simulink model "outdoor_weather_station"  (R2021b)
settings: Solver=VariableStepAuto  StartTime=0.0  StopTime=10.0  RelTol=1e-3
settings Model: Creator=solar  LastModifiedBy=solar

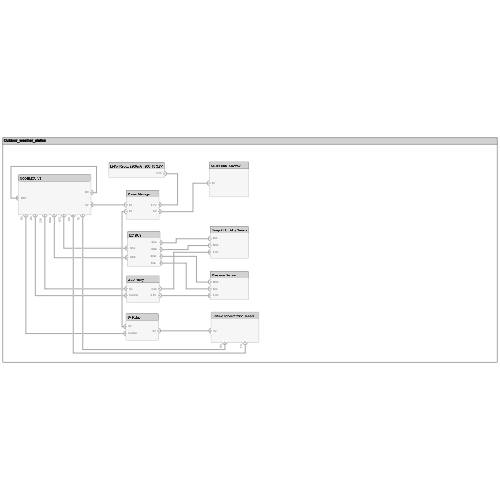
[thumbnail: Simulink's stored preview of the top-level diagram]
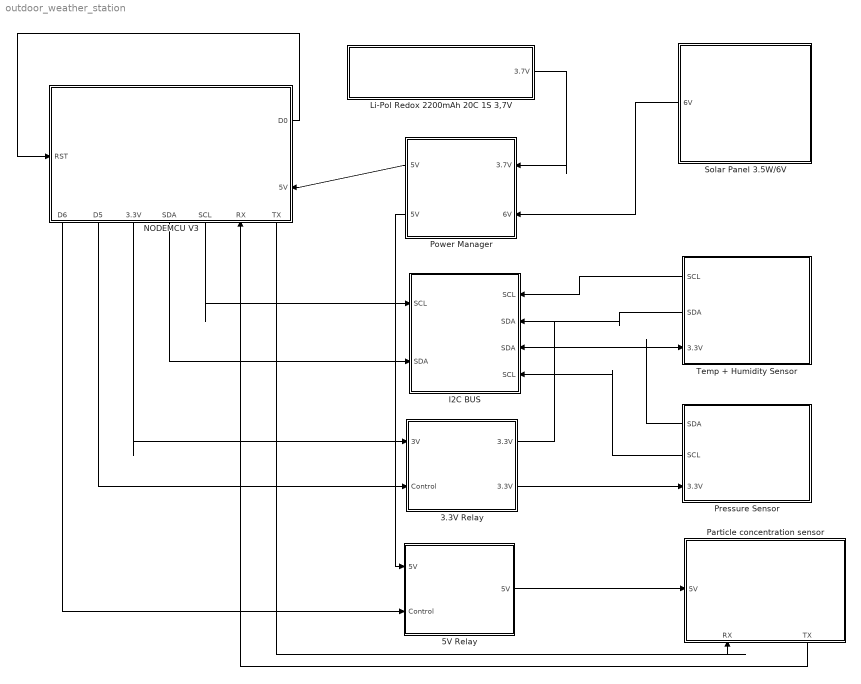
== system outdoor_weather_station ==
  3.3V Relay : Subsystem
      settings: PortSchema="{\"entries\":[{\"content\":{\"headerSize\":26,\"margin\":15,\"minimumSpacing\":25,\"sides\":[{\"content\":{\"connectorIds\":[\"In1\",\"In2\"]},\"type\":\"ConnectorPlacement.EquallySpacedRectSide\",\"uuid\":\"74d254f4-2ca4-49b7-9f78-a0cbae244880\"},{\"content\":{\"connectorIds\":[\"Out1\",\"Out2\"],\"side\":\"RIGHT\"},\"type\":\"ConnectorPlacement.EquallySpacedRectSide\",\"uuid\":\"e18b6892-bf0b-4da2-8b58-a37622c3cb9c\"},{\"content\":{\"connectorIds\":[],\"side\":\"TOP\"},\"type\":\"ConnectorPlacement.EquallySpacedRectSide\",\"uuid\":\"16187e55-be9e-4ec0-9bb4-e1bb1d52ffcb\"}]},\"type\":\"ConnectorPlacement.EquallySpacedConnector\",\"uuid\":\"64112707-4eaf-4f45-b3d2-d7f1b027a276\"}],\"packageUris\":[\"http://schema.mathworks.com/mf0/Connector/R2020b\"],\"version\":\"1.0\"}"
  5V Relay : Subsystem
      settings: PortSchema="{\"entries\":[{\"content\":{\"headerSize\":26,\"margin\":15,\"minimumSpacing\":25,\"sides\":[{\"content\":{\"connectorIds\":[\"In1\",\"In2\"]},\"type\":\"ConnectorPlacement.EquallySpacedRectSide\",\"uuid\":\"74d254f4-2ca4-49b7-9f78-a0cbae244880\"},{\"content\":{\"connectorIds\":[\"Out1\"],\"side\":\"RIGHT\"},\"type\":\"ConnectorPlacement.EquallySpacedRectSide\",\"uuid\":\"e18b6892-bf0b-4da2-8b58-a37622c3cb9c\"},{\"content\":{\"connectorIds\":[],\"side\":\"TOP\"},\"type\":\"ConnectorPlacement.EquallySpacedRectSide\",\"uuid\":\"16187e55-be9e-4ec0-9bb4-e1bb1d52ffcb\"}]},\"type\":\"ConnectorPlacement.EquallySpacedConnector\",\"uuid\":\"64112707-4eaf-4f45-b3d2-d7f1b027a276\"}],\"packageUris\":[\"http://schema.mathworks.com/mf0/Connector/R2020b\"],\"version\":\"1.0\"}"
  I2C BUS : Subsystem
      settings: PortSchema="{\"entries\":[{\"content\":{\"headerSize\":26,\"margin\":15,\"minimumSpacing\":25,\"sides\":[{\"content\":{\"connectorIds\":[\"In5\",\"In6\"]},\"type\":\"ConnectorPlacement.EquallySpacedRectSide\",\"uuid\":\"74d254f4-2ca4-49b7-9f78-a0cbae244880\"},{\"content\":{\"connectorIds\":[\"In1\",\"In2\",\"In3\",\"In4\"],\"side\":\"RIGHT\"},\"type\":\"ConnectorPlacement.EquallySpacedRectSide\",\"uuid\":\"e18b6892-bf0b-4da2-8b58-a37622c3cb9c\"},{\"content\":{\"connectorIds\":[],\"side\":\"TOP\"},\"type\":\"ConnectorPlacement.EquallySpacedRectSide\",\"uuid\":\"16187e55-be9e-4ec0-9bb4-e1bb1d52ffcb\"}]},\"type\":\"ConnectorPlacement.EquallySpacedConnector\",\"uuid\":\"64112707-4eaf-4f45-b3d2-d7f1b027a276\"}],\"packageUris\":[\"http://schema.mathworks.com/mf0/Connector/R2020b\"],\"version\":\"1.0\"}"
  "Li-Pol Redox 2200mAh 20C 1S 3,7V " : Subsystem
      settings: PortSchema="{\"entries\":[{\"content\":{\"headerSize\":26,\"margin\":15,\"minimumSpacing\":25,\"sides\":[{\"content\":{\"connectorIds\":[]},\"type\":\"ConnectorPlacement.EquallySpacedRectSide\",\"uuid\":\"74d254f4-2ca4-49b7-9f78-a0cbae244880\"},{\"content\":{\"connectorIds\":[\"Out1\"],\"side\":\"RIGHT\"},\"type\":\"ConnectorPlacement.EquallySpacedRectSide\",\"uuid\":\"e18b6892-bf0b-4da2-8b58-a37622c3cb9c\"},{\"content\":{\"connectorIds\":[],\"side\":\"TOP\"},\"type\":\"ConnectorPlacement.EquallySpacedRectSide\",\"uuid\":\"16187e55-be9e-4ec0-9bb4-e1bb1d52ffcb\"}]},\"type\":\"ConnectorPlacement.EquallySpacedConnector\",\"uuid\":\"64112707-4eaf-4f45-b3d2-d7f1b027a276\"}],\"packageUris\":[\"http://schema.mathworks.com/mf0/Connector/R2020b\"],\"version\":\"1.0\"}"
  NODEMCU V3 : Subsystem
      settings: PortSchema="{\"entries\":[{\"content\":{\"headerSize\":26,\"margin\":15,\"minimumSpacing\":25,\"sides\":[{\"content\":{\"connectorIds\":[\"In1\"]},\"type\":\"ConnectorPlacement.EquallySpacedRectSide\",\"uuid\":\"74d254f4-2ca4-49b7-9f78-a0cbae244880\"},{\"content\":{\"connectorIds\":[\"Out1\",\"In3\"],\"side\":\"RIGHT\"},\"type\":\"ConnectorPlacement.EquallySpacedRectSide\",\"uuid\":\"e18b6892-bf0b-4da2-8b58-a37622c3cb9c\"},{\"content\":{\"connectorIds\":[],\"side\":\"TOP\"},\"type\":\"ConnectorPlacement.EquallySpacedRectSide\",\"uuid\":\"16187e55-be9e-4ec0-9bb4-e1bb1d52ffcb\"},{\"content\":{\"connectorIds\":[\"Out3\",\"Out4\",\"Out5\",\"Out6\",\"Out7\",\"In2\",\"Out2\"],\"side\":\"BOTTOM\"},\"type\":\"ConnectorPlacement.EquallySpacedRectSide\",\"uuid\":\"a1eda6a0-5d0a-4f58-94a6-180de6326dd1\"}]},\"type\":\"ConnectorPlacement.EquallySpacedConnector\",\"uuid\":\"64112707-4eaf-4f45-b3d2-d7f1b027a276\"}],\"packageUris\":[\"http://schema.mathworks.com/mf0/Connector/R2020b\"],\"version\":\"1.0\"}"
  "Particle concentration sensor " : Subsystem
      settings: PortSchema="{\"entries\":[{\"content\":{\"headerSize\":26,\"margin\":15,\"minimumSpacing\":25,\"sides\":[{\"content\":{\"connectorIds\":[\"In2\"]},\"type\":\"ConnectorPlacement.EquallySpacedRectSide\",\"uuid\":\"74d254f4-2ca4-49b7-9f78-a0cbae244880\"},{\"content\":{\"connectorIds\":[],\"side\":\"RIGHT\"},\"type\":\"ConnectorPlacement.EquallySpacedRectSide\",\"uuid\":\"e18b6892-bf0b-4da2-8b58-a37622c3cb9c\"},{\"content\":{\"connectorIds\":[],\"side\":\"TOP\"},\"type\":\"ConnectorPlacement.EquallySpacedRectSide\",\"uuid\":\"16187e55-be9e-4ec0-9bb4-e1bb1d52ffcb\"},{\"content\":{\"connectorIds\":[\"In1\",\"Out1\"],\"side\":\"BOTTOM\"},\"type\":\"ConnectorPlacement.EquallySpacedRectSide\",\"uuid\":\"4097640e-2ff4-4c36-9601-de1d7640b3ef\"}]},\"type\":\"ConnectorPlacement.EquallySpacedConnector\",\"uuid\":\"64112707-4eaf-4f45-b3d2-d7f1b027a276\"}],\"packageUris\":[\"http://schema.mathworks.com/mf0/Connector/R2020b\"],\"version\":\"1.0\"}"
  Power Manager : Subsystem
      settings: PortSchema="{\"entries\":[{\"content\":{\"headerSize\":26,\"margin\":15,\"minimumSpacing\":25,\"sides\":[{\"content\":{\"connectorIds\":[\"Out2\",\"Out1\"]},\"type\":\"ConnectorPlacement.EquallySpacedRectSide\",\"uuid\":\"74d254f4-2ca4-49b7-9f78-a0cbae244880\"},{\"content\":{\"connectorIds\":[\"In1\",\"In2\"],\"side\":\"RIGHT\"},\"type\":\"ConnectorPlacement.EquallySpacedRectSide\",\"uuid\":\"e18b6892-bf0b-4da2-8b58-a37622c3cb9c\"},{\"content\":{\"connectorIds\":[],\"side\":\"TOP\"},\"type\":\"ConnectorPlacement.EquallySpacedRectSide\",\"uuid\":\"16187e55-be9e-4ec0-9bb4-e1bb1d52ffcb\"}]},\"type\":\"ConnectorPlacement.EquallySpacedConnector\",\"uuid\":\"64112707-4eaf-4f45-b3d2-d7f1b027a276\"}],\"packageUris\":[\"http://schema.mathworks.com/mf0/Connector/R2020b\"],\"version\":\"1.0\"}"
  "Pressure Sensor " : Subsystem
      settings: PortSchema="{\"entries\":[{\"content\":{\"headerSize\":26,\"margin\":15,\"minimumSpacing\":25,\"sides\":[{\"content\":{\"connectorIds\":[\"Out2\",\"Out1\",\"In1\"]},\"type\":\"ConnectorPlacement.EquallySpacedRectSide\",\"uuid\":\"74d254f4-2ca4-49b7-9f78-a0cbae244880\"},{\"content\":{\"connectorIds\":[],\"side\":\"RIGHT\"},\"type\":\"ConnectorPlacement.EquallySpacedRectSide\",\"uuid\":\"e18b6892-bf0b-4da2-8b58-a37622c3cb9c\"},{\"content\":{\"connectorIds\":[],\"side\":\"TOP\"},\"type\":\"ConnectorPlacement.EquallySpacedRectSide\",\"uuid\":\"16187e55-be9e-4ec0-9bb4-e1bb1d52ffcb\"}]},\"type\":\"ConnectorPlacement.EquallySpacedConnector\",\"uuid\":\"64112707-4eaf-4f45-b3d2-d7f1b027a276\"}],\"packageUris\":[\"http://schema.mathworks.com/mf0/Connector/R2020b\"],\"version\":\"1.0\"}"
  Solar Panel 3.5W/6V : Subsystem
      settings: PortSchema="{\"entries\":[{\"content\":{\"headerSize\":26,\"margin\":15,\"minimumSpacing\":25,\"sides\":[{\"content\":{\"connectorIds\":[\"Out1\"]},\"type\":\"ConnectorPlacement.EquallySpacedRectSide\",\"uuid\":\"74d254f4-2ca4-49b7-9f78-a0cbae244880\"},{\"content\":{\"connectorIds\":[],\"side\":\"RIGHT\"},\"type\":\"ConnectorPlacement.EquallySpacedRectSide\",\"uuid\":\"e18b6892-bf0b-4da2-8b58-a37622c3cb9c\"},{\"content\":{\"connectorIds\":[],\"side\":\"TOP\"},\"type\":\"ConnectorPlacement.EquallySpacedRectSide\",\"uuid\":\"16187e55-be9e-4ec0-9bb4-e1bb1d52ffcb\"}]},\"type\":\"ConnectorPlacement.EquallySpacedConnector\",\"uuid\":\"64112707-4eaf-4f45-b3d2-d7f1b027a276\"}],\"packageUris\":[\"http://schema.mathworks.com/mf0/Connector/R2020b\"],\"version\":\"1.0\"}"
  Temp + Humidity Sensor : Subsystem
      settings: PortSchema="{\"entries\":[{\"content\":{\"headerSize\":26,\"margin\":15,\"minimumSpacing\":25,\"sides\":[{\"content\":{\"connectorIds\":[\"Out2\",\"Out1\",\"In1\"]},\"type\":\"ConnectorPlacement.EquallySpacedRectSide\",\"uuid\":\"74d254f4-2ca4-49b7-9f78-a0cbae244880\"},{\"content\":{\"connectorIds\":[],\"side\":\"RIGHT\"},\"type\":\"ConnectorPlacement.EquallySpacedRectSide\",\"uuid\":\"e18b6892-bf0b-4da2-8b58-a37622c3cb9c\"},{\"content\":{\"connectorIds\":[],\"side\":\"TOP\"},\"type\":\"ConnectorPlacement.EquallySpacedRectSide\",\"uuid\":\"16187e55-be9e-4ec0-9bb4-e1bb1d52ffcb\"}]},\"type\":\"ConnectorPlacement.EquallySpacedConnector\",\"uuid\":\"64112707-4eaf-4f45-b3d2-d7f1b027a276\"}],\"packageUris\":[\"http://schema.mathworks.com/mf0/Connector/R2020b\"],\"version\":\"1.0\"}"
  wires:
  Solar Panel 3.5W/6V/1(6V) -> Power Manager/2(6V)
  Power Manager/2(5V) -> NODEMCU V3/3(5V)
  "Li-Pol Redox 2200mAh 20C 1S 3,7V "/1(3.7V) -> Power Manager/1(3.7V)
  NODEMCU V3/7(SCL) -> I2C BUS/5(SCL)
  NODEMCU V3/6(SDA) -> I2C BUS/6(SDA)
  NODEMCU V3/4(D5) -> 3.3V Relay/2(Control)
  NODEMCU V3/3(D6) -> 5V Relay/2(Control)
  3.3V Relay/1(3.3V) -> Temp + Humidity Sensor/1(3.3V)
  Temp + Humidity Sensor/2(SCL) -> I2C BUS/1("SCL ")
  Temp + Humidity Sensor/1(SDA) -> I2C BUS/2("SDA ")
  3.3V Relay/2("3.3V ") -> "Pressure Sensor "/1("3.3V ")
  "Pressure Sensor "/1("SCL  ") -> I2C BUS/4("SCL  ")
  "Pressure Sensor "/2("SDA  ") -> I2C BUS/3("SDA  ")
  5V Relay/1(5V) -> "Particle concentration sensor "/2(5V)
  NODEMCU V3/5("3.3V ") -> 3.3V Relay/1(3V)
  Power Manager/1("5V  ") -> 5V Relay/1("5V  ")
  NODEMCU V3/2(TX) -> "Particle concentration sensor "/1(RX)
  "Particle concentration sensor "/1(TX) -> NODEMCU V3/2(RX)
  NODEMCU V3/1(D0) -> NODEMCU V3/1(RST)

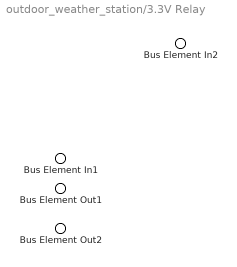
== system outdoor_weather_station/3.3V Relay ==
  Bus Element In2 : Inport  PortName=3V
  Bus Element In1 : Inport  Port=2  PortName=Control
  Bus Element Out1 : Outport  PortName=3.3V
  Bus Element Out2 : Outport  Port=2  PortName=3.3V

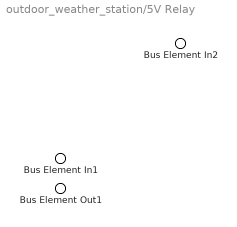
== system outdoor_weather_station/5V Relay ==
  Bus Element In2 : Inport  PortName=5V
  Bus Element In1 : Inport  Port=2  PortName=Control
  Bus Element Out1 : Outport  PortName=5V

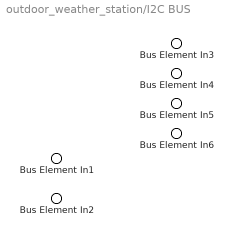
== system outdoor_weather_station/I2C BUS ==
  Bus Element In3 : Inport  PortName=SCL
  Bus Element In4 : Inport  Port=2  PortName=SDA
  Bus Element In6 : Inport  Port=3  PortName=SDA
  Bus Element In5 : Inport  Port=4  PortName=SCL
  Bus Element In1 : Inport  Port=5  PortName=SCL
  Bus Element In2 : Inport  Port=6  PortName=SDA

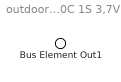
== system outdoor_weather_station/Li-Pol Redox 2200mAh 20C 1S 3,7V  ==
  Bus Element Out1 : Outport  PortName=3.7V

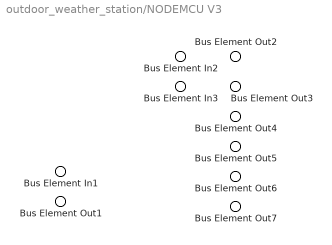
== system outdoor_weather_station/NODEMCU V3 ==
  Bus Element In3 : Inport  PortName=RST
  Bus Element In2 : Inport  Port=2  PortName=RX
  Bus Element In1 : Inport  Port=3  PortName=5V
  Bus Element Out7 : Outport  PortName=D0
  Bus Element Out6 : Outport  Port=2  PortName=TX
  Bus Element Out4 : Outport  Port=3  PortName=D6
  Bus Element Out3 : Outport  Port=4  PortName=D5
  Bus Element Out5 : Outport  Port=5  PortName=3.3V
  Bus Element Out2 : Outport  Port=6  PortName=SDA
  Bus Element Out1 : Outport  Port=7  PortName=SCL

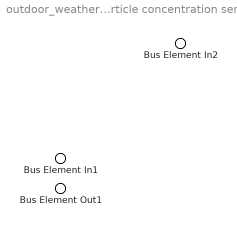
== system outdoor_weather_station/Particle concentration sensor  ==
  Bus Element In2 : Inport  PortName=RX
  Bus Element In1 : Inport  Port=2  PortName=5V
  Bus Element Out1 : Outport  PortName=TX

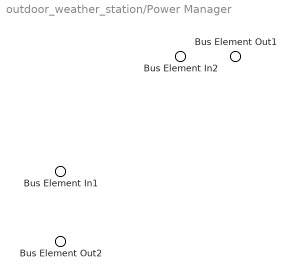
== system outdoor_weather_station/Power Manager ==
  Bus Element In2 : Inport  PortName=3.7V
  Bus Element In1 : Inport  Port=2  PortName=6V
  Bus Element Out1 : Outport  PortName=5V
  Bus Element Out2 : Outport  Port=2  PortName=5V

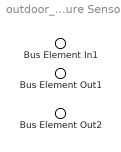
== system outdoor_weather_station/Pressure Sensor  ==
  Bus Element In1 : Inport  PortName=3.3V
  Bus Element Out1 : Outport  PortName=SCL
  Bus Element Out2 : Outport  Port=2  PortName=SDA

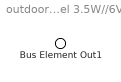
== system outdoor_weather_station/Solar Panel 3.5W//6V ==
  Bus Element Out1 : Outport  PortName=6V

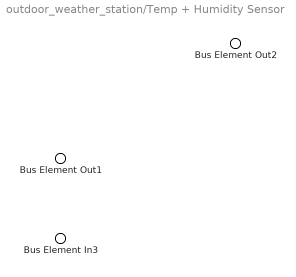
== system outdoor_weather_station/Temp + Humidity Sensor ==
  Bus Element In3 : Inport  PortName=3.3V
  Bus Element Out2 : Outport  PortName=SDA
  Bus Element Out1 : Outport  Port=2  PortName=SCL
